simulink model "rtwdemo_lmsadeq"  (Simulink 6.0)
settings: Solver=FixedStepDiscrete  SolverMode=SingleTasking  StartTime=0.0  StopTime=1000  RelTol=1e-3  AbsTol=1e-6
libraries: simulink x2, dspsnks4 x2, rtwdemowidgets x1, dspsigops x1, dsparch4 x1, dspsigattribs x1, dspadpt3 x1
settings Model: RequirementInfo=9  CovMetricSettings=d  Creator=The MathWorks Inc.  LastModifiedBy=batserve  ExtModeTrigMode=oneshot  ExtModeArmWhenConnect=off  ExtModeAutoUpdateStatusClock=off
settings DataIOCC: LimitDataPoints=off  SaveOutput=off  SaveTime=off  SignalLoggingName=sigsOut
settings OptimizationCC: InlineParams=on  EnforceIntegerDowncast=off  StateBitsets=on  DataBitsets=on  UseTempVars=on
settings DebuggingCC: CheckExecutionContextPreStartOutputMsg=on  CheckExecutionContextRuntimeOutputMsg=on  SolverPrmCheckMsg=none  IntegerOverflowMsg=none
settings RTWCC: TLCOptions=-p0 -aWarnNonSaturatedBlocks=0  GenerateReport=on  RTWVerbose=off  ProcessScript=grt_make_rtw_hook  LaunchReport=on
settings CodeAppCC: ForceParamTrailComments=on
settings GRTTargetCC: MatFileLogging=off

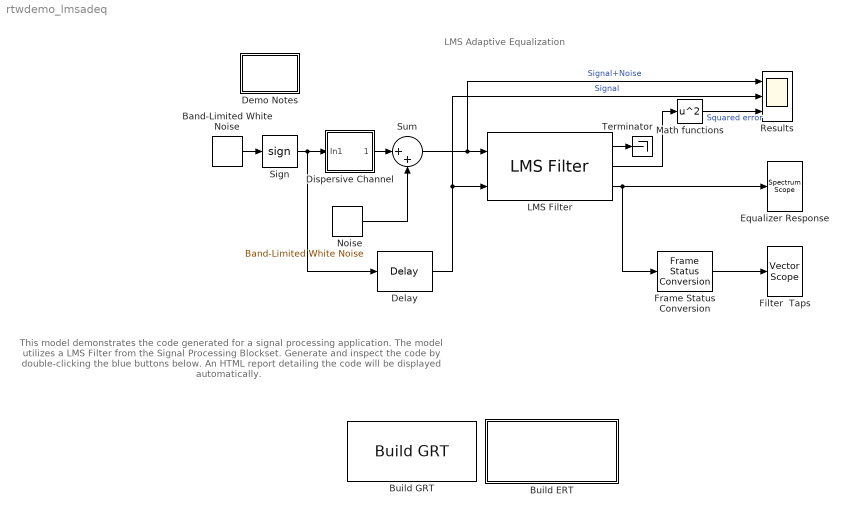
== system rtwdemo_lmsadeq ==
  note: LMS Adaptive Equalization
  note: This model demonstrates the code generated for a signal processing application.
      | The model utilizes a LMS Filter from the Signal Processing Blockset.
      |
      | Generate and inspect the code by double-clicking the blue buttons below.  An
      | HTML report detailing the code will be displayed automatically.
  Band-Limited White Noise : simulink/Sources/Band-Limited White Noise  Cov=1e-5  Ts=1e-5  seed=12345
  Build ERT : Subsystem  AncestorBlock=rtwdemowidgets/Build ERT  PropExecContextAcrossSSBoundary=on  mask{attrib_overrides={}}
      mask prompts: attrib_overrides "List of attributes to preserve (cell of strings):"
      mask help: Enter the attributes of the configuration set that you want preserved. Otherwise, the default configuration script will override your current settings.
      settings: OpenFcn=|
      | model=bdroot;
      | overrides=get_param(gcb,'attrib_overrides');
      | try
      |   rtwconfiguredemo(model,'noop',false,overrides);
      |   cs = getActiveConfigSet(model);
      |   set_param(cs,'SupportComplex','on');
      |   rtwbuilddemomodel(model);
      | catch
      |   error(lasterr);
      | end
      mask Display:
      | disp(['Generate Code Using\n',...
      | 	  'Real-Time Workshop\n',...
      | 	  'Embedded Coder\n'...
      | 	  '(double-click)'])
  Build GRT : rtwdemowidgets/Build GRT  attrib_overrides={}
  Delay : dspsigops/Delay  dly_unit=Samples  delay=6  ic_detail=off  dif_ic_for_ch=off  dif_ic_for_dly=off  ic=0  reset_popup=None
  Demo Notes : Subsystem  PropExecContextAcrossSSBoundary=on
      mask Display: disp('Demo\nNotes')
  Dispersive Channel : Subsystem  PropExecContextAcrossSSBoundary=on  mask(Simple Dispersive Channel){d=3.5}
      mask prompts: d "Dispersion:"
      mask help: Dispersive channel filter.
      mask init:
      | b=.5*(1+cos(2*pi./d.*[-1 0 1])); h=log(abs(freqz(b,1,64)));
      mask Help: Dispersive channel filter
      mask Display: plot(h)
  Equalizer Response : dspsnks4/Spectrum Scope  ScopeProperties=on  Domain=Frequency  HorizSpan=1  UseBuffer=off  BufferSize=128  Overlap=64  inpFftLenInherit=on  FFTlength=128  numAvg=2  DisplayProperties=off  AxisGrid=on  Memory=off  FrameNumber=off  AxisLegend=off  AxisZoom=off  OpenScopeAtSimStart=on  OpenScopeImmediately=off  FigPos=[29 124 450 360]  AxisProperties=off  XUnits=Hertz  XRange=[0...Fs/2]  InheritXIncr=on  XIncr=1  XLabel=Samples  YUnits=dB  YLabel=Magnitude, dB  LineProperties=off
      settings: YMin=-12  YMax=8
  Filter  Taps : dspsnks4/Vector Scope  ScopeProperties=on  Domain=User-defined  HorizSpan=1  DisplayProperties=off  AxisGrid=on  Memory=off  FrameNumber=off  AxisLegend=off  AxisZoom=off  OpenScopeAtSimStart=on  OpenScopeImmediately=off  FigPos=[491 123 450 360]  AxisProperties=off  XUnits=Hertz  XRange=[0...Fs/2]  InheritXIncr=off  XIncr=1  XLabel=Samples  YUnits=dB  YLabel=Equalizer Coefficients  LineProperties=off  LineMarkers=.
      settings: YMin=-1  YMax=2
  Frame Status Conversion : dspsigattribs/Frame Status Conversion  growRefPort=off  outframe=Frame-based
  LMS Filter : dspadpt3/LMS Filter  DialogController=dspDDGCreate  DialogControllerArgs=DataTag1  Algo=Normalized LMS  L=11  stepflag=Dialog  mu=0.5  leakage=1.0  ic=0  Adapt=off  resetflag=None  weights=on  secondCoeffMode=User-defined  secondCoeffWordLength=2  secondCoeffFracLength=15  accum2Mode=User-defined  accum2FracLength=20  prodOutput2Mode=User-defined  prodOutput2FracLength=20  prodOutput3Mode=User-defined  prodOutput3FracLength=20  prodOutput4Mode=User-defined  prodOutput4FracLength=20  quotientMode=User-defined  quotientFracLength=20  roundingMode=Floor  overflowMode=off  addnparflag=off
  Math functions : Math  Operator=square  SaturateOnIntegerOverflow=on
  Noise : simulink/Sources/Band-Limited White Noise  Cov=.002e-5  Ts=1e-5  seed=[23341]
  Results : Scope  NumInputPorts=3
      settings: TimeRange=0.005  YMin=-2~0~0  YMax=2~2~1  DataFormat=Array
  Sign : Signum
  Sum : Sum  Inputs=|++  SaturateOnIntegerOverflow=on  InputSameDT=on
  Terminator : Terminator
  wires:
  LMS Filter/3 -> Frame Status Conversion/1, Equalizer Response/1
  Dispersive Channel/1(Out1) -> Sum/1
  Band-Limited White Noise/1 -> Sign/1
  Noise/1 -> Sum/2
  Sign/1 -> Dispersive Channel/1(In1), Delay/1
  LMS Filter/2 -> Math functions/1
  Math functions/1 -> Results/3  "Squared error"
  Delay/1 -> LMS Filter/2, Results/2  "Signal"
  Frame Status Conversion/1 -> Filter  Taps/1
  LMS Filter/1 -> Terminator/1
  Sum/1 -> LMS Filter/1, Results/1  "Signal+Noise"

== system rtwdemo_lmsadeq/Build ERT ==

== system rtwdemo_lmsadeq/Demo Notes ==
  note: Adaptive Channel Equalization
      |
      | This demonstrates the ability of the LMS algorithm
      | to adaptively compute the estimate of an FIR
      | equalization filter.
      |
      | For more information on the LMS adaptive filter
      | or channel equalization, see
      | S. Haykin, "Adaptive Filter Theory",
      | 3rd Ed., Prentice Hall, 1996.

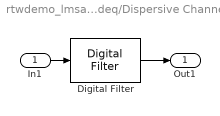
== system rtwdemo_lmsadeq/Dispersive Channel ==
  In1 : Inport  Port=1  LatchInput=off
  Digital Filter : dsparch4/Digital Filter  DialogController=dspDDGCreate  DialogControllerArgs=DataTag0  TypePopup=FIR (all zeros)  IIRFiltStruct=Direct form II transposed  AllPoleFiltStruct=Direct form  FIRFiltStruct=Direct form  CoeffSource=Specify via dialog  NumCoeffs=b  DenCoeffs=[1 0.1]  BiQuadCoeffs=[1 0.3 0.4 1 0.1 0.2]  LatticeCoeffs=[0.2 0.4]  denIgnore=on  FiltPerSampPopup=One filter per frame  IC=0  ICnum=0  ICden=0  roundingMode=Floor  overflowMode=off  ScaleValues=1  scaleValueFracLength=14  stageInFracLength=15  stageOutFracLength=15
  Out1 : Outport
  wires:
  Digital Filter/1 -> Out1/1
  In1/1 -> Digital Filter/1
